simulink model "mainModel"  (R2025b)
settings: Solver=ode1  StartTime=0.0  StopTime=meas.u_alpha.time(end)  FixedStep=0.001  RelTol=1e-3
values from neighbouring files (symbols this model uses):
  alpha0 = params(1)    [Throttle_Parameter_Identification.m]
  alpha1 = params(2)    [Throttle_Parameter_Identification.m]
  R = 287    [Throttle_Parameter_Identification.m]
undefined symbols (not defined in the file or in its folder): beta0, gamma0, gamma1, H_l, k_eta, kappa, lambda, meas, nu0, nu1, nu_gen, sigma0, theta_e, Vc, Vd, Vm
settings Model: Creator=khanh  LastModifiedBy=khanh

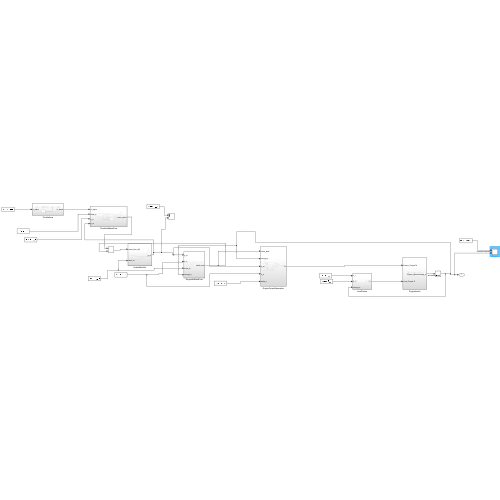
[thumbnail: Simulink's stored preview of the top-level diagram]
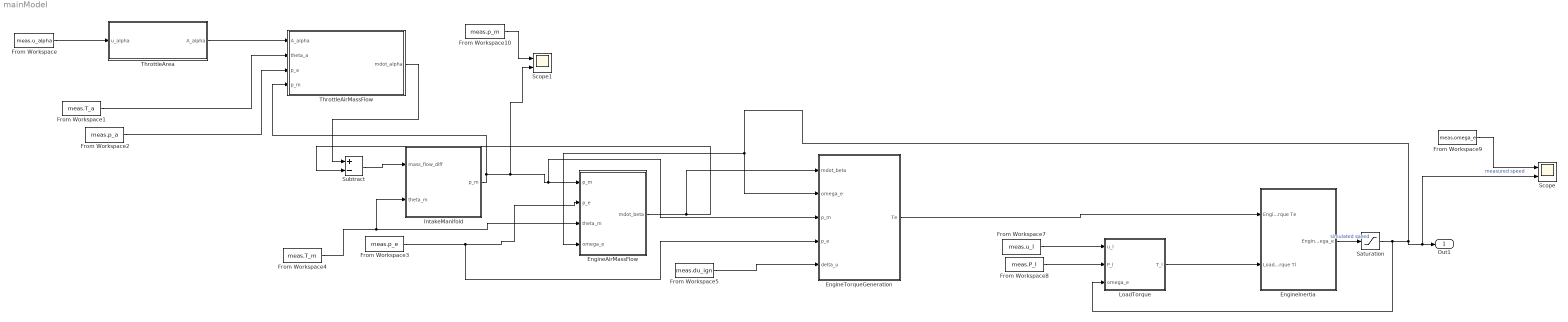
== system mainModel ==
  EngineAirMassFlow : Subsystem
  EngineInertia : Subsystem
  EngineTorqueGeneration : Subsystem
  From Workspace : FromWorkspace  VariableName=meas.u_alpha
  From Workspace1 : FromWorkspace  VariableName=meas.T_a
  From Workspace10 : FromWorkspace  VariableName=meas.p_m
  From Workspace2 : FromWorkspace  VariableName=meas.p_a
  From Workspace3 : FromWorkspace  VariableName=meas.p_e
  From Workspace4 : FromWorkspace  VariableName=meas.T_m
  From Workspace5 : FromWorkspace  VariableName=meas.du_ign
  From Workspace7 : FromWorkspace  VariableName=meas.u_l
  From Workspace8 : FromWorkspace  VariableName=meas.P_l
  From Workspace9 : FromWorkspace  VariableName=meas.omega_e
  IntakeManifold : Subsystem
  LoadTorque : Subsystem
  Saturation : Saturate  UpperLimit=500  LowerLimit=20
  Scope : Scope  NumInputPorts=2
      settings: ActiveDisplayYMinimum=-152.23064174316474  ActiveDisplayYMaximum=346.81367867125368
  Scope1 : Scope  NumInputPorts=2
      settings: ActiveDisplayYMinimum=10127.672299605907  ActiveDisplayYMaximum=44236.443903132655  DataLoggingVariableName=ScopeData4
  Subtract : Sum  Inputs=+-
  ThrottleAirMassFlow : Subsystem
  ThrottleArea : Subsystem
  Out1 : Outport
  wires:
  From Workspace2/1 -> ThrottleAirMassFlow/3(p_a)
  EngineAirMassFlow/1(mdot_beta) -> EngineTorqueGeneration/1(mdot_beta), Subtract/2
  From Workspace3/1 -> EngineTorqueGeneration/4(p_e), EngineAirMassFlow/2(p_e)
  From Workspace1/1 -> ThrottleAirMassFlow/2(theta_a)
  From Workspace4/1 -> EngineAirMassFlow/3(theta_m), IntakeManifold/2(theta_m)
  From Workspace/1 -> ThrottleArea/1(u_alpha)
  ThrottleArea/1(A_alpha) -> ThrottleAirMassFlow/1(A_alpha)
  ThrottleAirMassFlow/1(mdot_alpha) -> Subtract/1
  Saturation/1 -> LoadTorque/3(omega_e), Scope/2, Out1/1, EngineAirMassFlow/4(omega_e), EngineTorqueGeneration/2(omega_e)
  From Workspace9/1 -> Scope/1  "measured speed"
  LoadTorque/1(T_l) -> EngineInertia/2(Load_Torque Tl)
  From Workspace10/1 -> Scope1/1
  EngineTorqueGeneration/1(Te) -> EngineInertia/1(Engine_Torque Te)
  From Workspace7/1 -> LoadTorque/1(u_l)
  EngineInertia/1(Engine_Speed omega_e) -> Saturation/1  "simulated speed"
  Subtract/1 -> IntakeManifold/1(mass_flow_diff)
  From Workspace8/1 -> LoadTorque/2(P_l)
  From Workspace5/1 -> EngineTorqueGeneration/5(delta_u)
  IntakeManifold/1(p_m) -> ThrottleAirMassFlow/4(p_m), Scope1/2, EngineTorqueGeneration/3(p_m), EngineAirMassFlow/1(p_m)

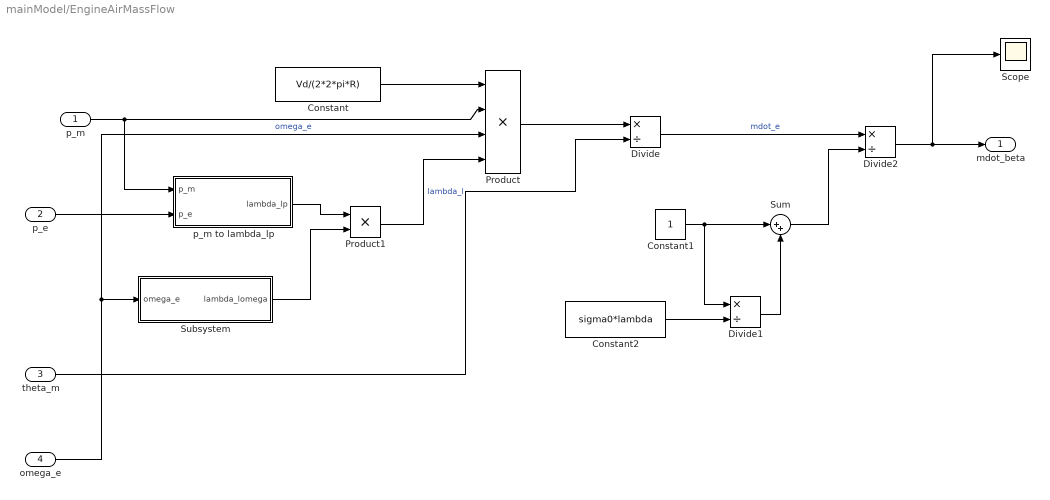
== system mainModel/EngineAirMassFlow ==
  p_m : Inport
  p_e : Inport  Port=2
  theta_m : Inport  Port=3
  omega_e : Inport  Port=4
  Constant : Constant  Value=Vd/(2*2*pi*R)
  Constant1 : Constant
  Constant2 : Constant  Value=sigma0*lambda
  Divide : Product  Inputs=*/
  Divide1 : Product  Inputs=*/
  Divide2 : Product  Inputs=*/
  Product : Product  Inputs=4
  Product1 : Product
  Scope : Scope
      settings: ActiveDisplayYMinimum=-1  ActiveDisplayYMaximum=1  DataLoggingVariableName=ScopeData3
  Subsystem : Subsystem
  Sum : Sum  Inputs=|++
  p_m to lambda_lp : Subsystem
  mdot_beta : Outport
  wires:
  Sum/1 -> Divide2/2
  Constant1/1 -> Divide1/1, Sum/1
  Divide/1 -> Divide2/1  "mdot_e"
  p_e/1 -> p_m to lambda_lp/2(p_e)
  Divide2/1 -> Scope/1, mdot_beta/1
  Constant/1 -> Product/1
  theta_m/1 -> Divide/2
  Product1/1 -> Product/4  "lambda_l"
  Constant2/1 -> Divide1/2
  omega_e/1 -> Product/3, Subsystem/1(omega_e)  "omega_e"
  Divide1/1 -> Sum/2
  p_m/1 -> p_m to lambda_lp/1(p_m), Product/2
  Product/1 -> Divide/1
  Subsystem/1(lambda_lomega) -> Product1/2
  p_m to lambda_lp/1(lambda_lp) -> Product1/1

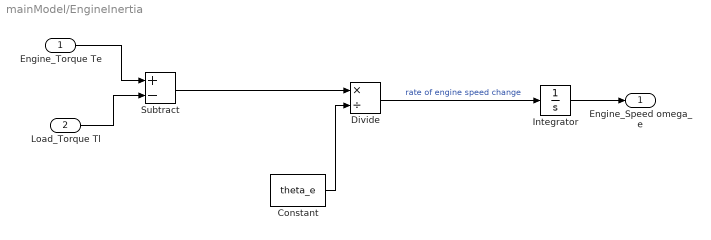
== system mainModel/EngineInertia ==
  Engine_Torque Te : Inport
  Load_Torque Tl : Inport  Port=2
  Constant : Constant  Value=theta_e
  Divide : Product  Inputs=*/
  Integrator : Integrator  InitialCondition=meas.omega_e.signals.values(1)
  Subtract : Sum  Inputs=+-
  Engine_Speed omega_e : Outport
  wires:
  Load_Torque Tl/1 -> Subtract/2
  Engine_Torque Te/1 -> Subtract/1
  Constant/1 -> Divide/2
  Divide/1 -> Integrator/1  "rate of engine speed change"
  Subtract/1 -> Divide/1
  Integrator/1 -> Engine_Speed omega_e/1

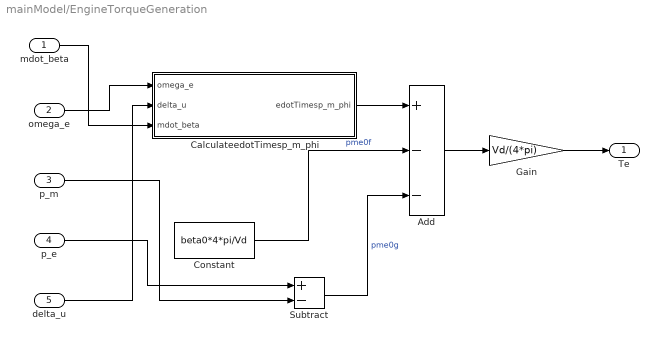
== system mainModel/EngineTorqueGeneration ==
  mdot_beta : Inport
  omega_e : Inport  Port=2
  p_m : Inport  Port=3
  p_e : Inport  Port=4
  delta_u : Inport  Port=5
  Add : Sum  Inputs=+--
  CalculateedotTimesp_m_phi : Subsystem
  Constant : Constant  Value=beta0*4*pi/Vd
  Gain : Gain  Gain=Vd/(4*pi)
  Subtract : Sum  Inputs=+-
  Te : Outport
  wires:
  Gain/1 -> Te/1
  Add/1 -> Gain/1
  Subtract/1 -> Add/3  "pme0g"
  p_m/1 -> Subtract/2
  delta_u/1 -> CalculateedotTimesp_m_phi/2(delta_u)
  CalculateedotTimesp_m_phi/1(edotTimesp_m_phi) -> Add/1
  mdot_beta/1 -> CalculateedotTimesp_m_phi/3(mdot_beta)
  Constant/1 -> Add/2  "pme0f"
  p_e/1 -> Subtract/1
  omega_e/1 -> CalculateedotTimesp_m_phi/1(omega_e)

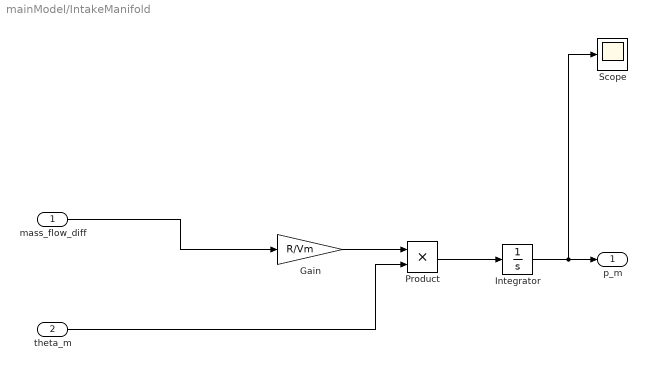
== system mainModel/IntakeManifold ==
  mass_flow_diff : Inport
  theta_m : Inport  Port=2
  Gain : Gain  Gain=R/Vm
  Integrator : Integrator  InitialCondition=meas.p_m.signals.values(1)
  Product : Product
  Scope : Scope
      settings: ActiveDisplayYMinimum=14149.965653298506  ActiveDisplayYMaximum=34149.96565329851  DataLoggingVariableName=ScopeData2
  p_m : Outport
  wires:
  Gain/1 -> Product/1
  Product/1 -> Integrator/1
  theta_m/1 -> Product/2
  Integrator/1 -> Scope/1, p_m/1
  mass_flow_diff/1 -> Gain/1

== system mainModel/LoadTorque ==
  u_l : Inport
  P_l : Inport  Port=2
  omega_e : Inport  Port=3
  Load Torque Subsystem : Subsystem
  T_l : Outport
  wires:
  P_l/1 -> Load Torque Subsystem/2(P_l)
  u_l/1 -> Load Torque Subsystem/1(u_l)
  omega_e/1 -> Load Torque Subsystem/3(omega_e)
  Load Torque Subsystem/1(Out1) -> T_l/1

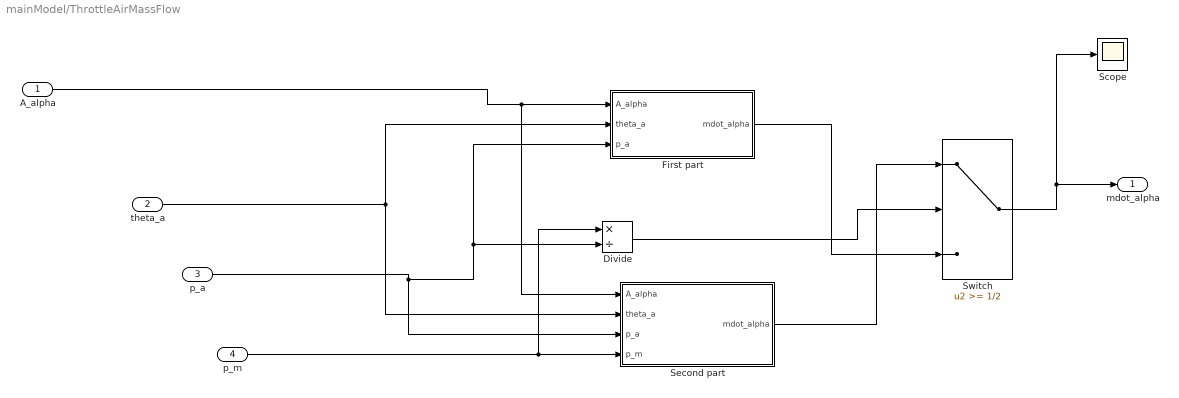
== system mainModel/ThrottleAirMassFlow ==
  A_alpha : Inport
  theta_a : Inport  Port=2
  p_a : Inport  Port=3
  p_m : Inport  Port=4
  Divide : Product  Inputs=*/
  First part : Subsystem
  Scope : Scope
      settings: ActiveDisplayYMinimum=-1  ActiveDisplayYMaximum=1
  "Second part " : Subsystem
  Switch : Switch  Threshold=1/2  SaturateOnIntegerOverflow=off  InputSameDT=off
  mdot_alpha : Outport
  wires:
  A_alpha/1 -> "Second part "/1(A_alpha), First part/1(A_alpha)
  p_a/1 -> "Second part "/3(p_a), First part/3(p_a), Divide/2
  p_m/1 -> "Second part "/4(p_m), Divide/1
  First part/1(mdot_alpha) -> Switch/3
  Switch/1 -> Scope/1, mdot_alpha/1
  Divide/1 -> Switch/2
  "Second part "/1(mdot_alpha) -> Switch/1
  theta_a/1 -> "Second part "/2(theta_a), First part/2(theta_a)

== system mainModel/ThrottleArea ==
  u_alpha : Inport
  Constant : Constant  Value=alpha0
  Gain : Gain  Gain=alpha1
  Sum : Sum  Inputs=|++
  A_alpha : Outport
  wires:
  Sum/1 -> A_alpha/1
  u_alpha/1 -> Gain/1
  Constant/1 -> Sum/2
  Gain/1 -> Sum/1

== system mainModel/EngineAirMassFlow/Subsystem ==
  omega_e : Inport
  Constant : Constant  Value=gamma0
  Gain : Gain  Gain=gamma1
  Sum : Sum  Inputs=|++
  lambda_lomega : Outport
  wires:
  Constant/1 -> Sum/1
  omega_e/1 -> Gain/1
  Gain/1 -> Sum/2
  Sum/1 -> lambda_lomega/1

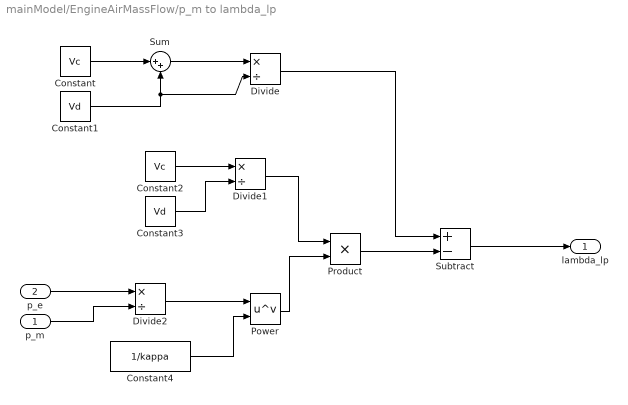
== system mainModel/EngineAirMassFlow/p_m to lambda_lp ==
  p_m : Inport
  p_e : Inport  Port=2
  Constant : Constant  Value=Vc
  Constant1 : Constant  Value=Vd
  Constant2 : Constant  Value=Vc
  Constant3 : Constant  Value=Vd
  Constant4 : Constant  Value=1/kappa
  Divide : Product  Inputs=*/
  Divide1 : Product  Inputs=*/
  Divide2 : Product  Inputs=*/
  Power : Math  Operator=pow
  Product : Product
  Subtract : Sum  Inputs=+-
  Sum : Sum  Inputs=|++
  lambda_lp : Outport
  wires:
  Constant/1 -> Sum/1
  Constant1/1 -> Sum/2, Divide/2
  Sum/1 -> Divide/1
  Constant2/1 -> Divide1/1
  Constant3/1 -> Divide1/2
  Divide2/1 -> Power/1
  Constant4/1 -> Power/2
  Divide1/1 -> Product/1
  Power/1 -> Product/2
  Divide/1 -> Subtract/1
  Product/1 -> Subtract/2
  Subtract/1 -> lambda_lp/1
  p_e/1 -> Divide2/1
  p_m/1 -> Divide2/2

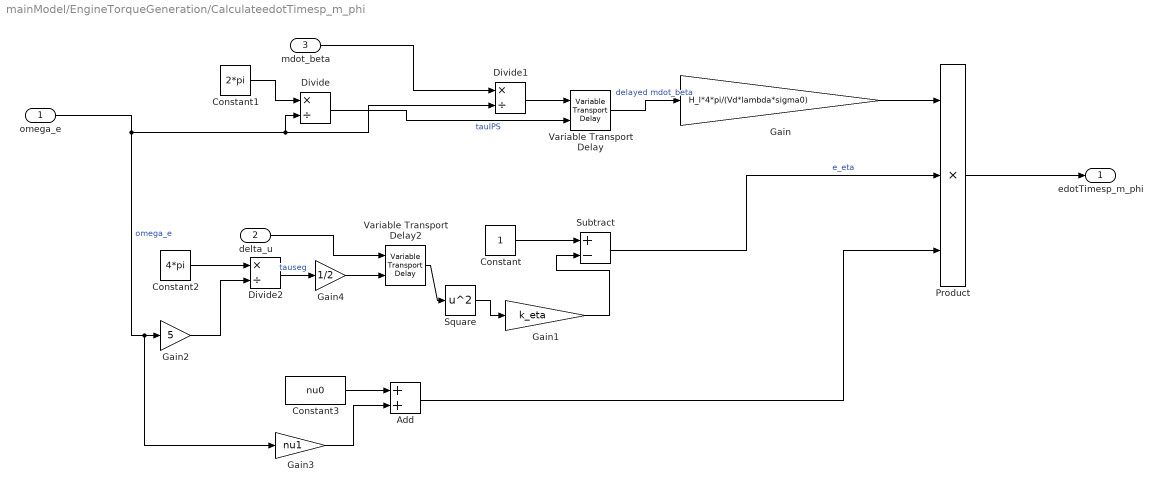
== system mainModel/EngineTorqueGeneration/CalculateedotTimesp_m_phi ==
  omega_e : Inport
  delta_u : Inport  Port=2
  mdot_beta : Inport  Port=3
  Add : Sum
  Constant : Constant
  Constant1 : Constant  Value=2*pi
  Constant2 : Constant  Value=4*pi
  Constant3 : Constant  Value=nu0
  Divide : Product  Inputs=*/
  Divide1 : Product  Inputs=*/
  Divide2 : Product  Inputs=*/
  Gain : Gain  Gain=H_l*4*pi/(Vd*lambda*sigma0)
  Gain1 : Gain  Gain=k_eta
  Gain2 : Gain  Gain=5
  Gain3 : Gain  Gain=nu1
  Gain4 : Gain  Gain=1/2
  Product : Product  Inputs=3
  Square : Math  Operator=square
  Subtract : Sum  Inputs=+-
  Variable Transport Delay : VariableTransportDelay  VariableDelayType=Variable transport delay  MaximumDelay=10
  Variable Transport Delay2 : VariableTransportDelay  VariableDelayType=Variable transport delay  MaximumDelay=10
  edotTimesp_m_phi : Outport
  wires:
  Constant/1 -> Subtract/1
  Gain1/1 -> Subtract/2
  Subtract/1 -> Product/2  "e_eta"
  omega_e/1 -> Gain3/1, Gain2/1, Divide1/2, Divide/2  "omega_e"
  Constant1/1 -> Divide/1
  Constant2/1 -> Divide2/1
  Gain2/1 -> Divide2/2
  Divide2/1 -> Gain4/1  "tauseg"
  delta_u/1 -> Variable Transport Delay2/1
  Constant3/1 -> Add/1
  Gain3/1 -> Add/2
  Gain/1 -> Product/1
  Add/1 -> Product/3
  Product/1 -> edotTimesp_m_phi/1
  Divide/1 -> Variable Transport Delay/2  "tauIPS"
  mdot_beta/1 -> Divide1/1
  Divide1/1 -> Variable Transport Delay/1
  Variable Transport Delay/1 -> Gain/1  "delayed mdot_beta"
  Variable Transport Delay2/1 -> Square/1
  Square/1 -> Gain1/1
  Gain4/1 -> Variable Transport Delay2/2

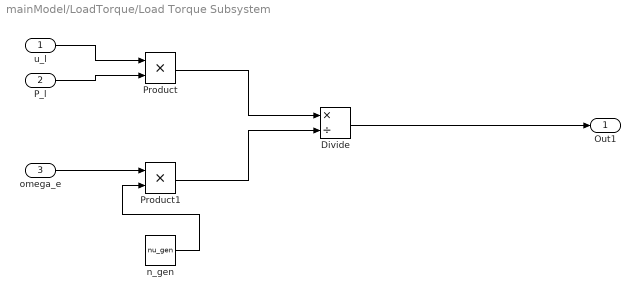
== system mainModel/LoadTorque/Load Torque Subsystem ==
  u_l : Inport
  P_l : Inport  Port=2
  omega_e : Inport  Port=3
  Divide : Product  Inputs=*/
  Product : Product
  Product1 : Product
  n_gen : Constant  Value=nu_gen
  Out1 : Outport
  wires:
  P_l/1 -> Product/2
  u_l/1 -> Product/1
  omega_e/1 -> Product1/1
  n_gen/1 -> Product1/2
  Divide/1 -> Out1/1
  Product/1 -> Divide/1
  Product1/1 -> Divide/2

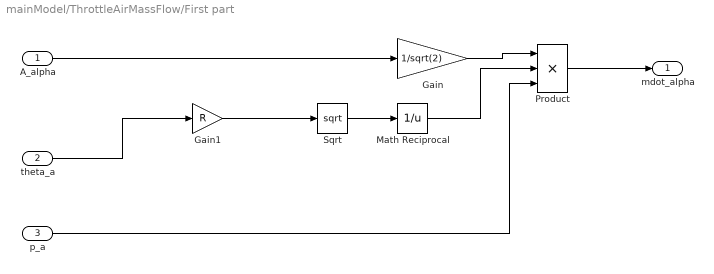
== system mainModel/ThrottleAirMassFlow/First part ==
  A_alpha : Inport
  theta_a : Inport  Port=2
  p_a : Inport  Port=3
  Gain : Gain  Gain=1/sqrt(2)
  Gain1 : Gain  Gain=R
  Math Reciprocal : Math  Operator=reciprocal  SignedPower=on
  Product : Product  Inputs=3
  Sqrt : Sqrt
  mdot_alpha : Outport
  wires:
  Sqrt/1 -> Math Reciprocal/1
  p_a/1 -> Product/3
  Gain/1 -> Product/1
  Gain1/1 -> Sqrt/1
  theta_a/1 -> Gain1/1
  Product/1 -> mdot_alpha/1
  A_alpha/1 -> Gain/1
  Math Reciprocal/1 -> Product/2

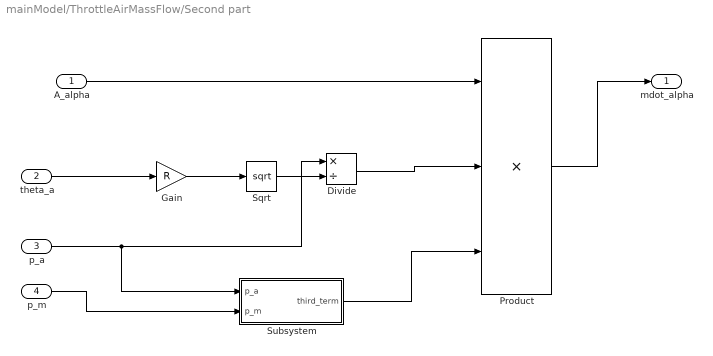
== system mainModel/ThrottleAirMassFlow/Second part  ==
  A_alpha : Inport
  theta_a : Inport  Port=2
  p_a : Inport  Port=3
  p_m : Inport  Port=4
  Divide : Product  Inputs=*/
  Gain : Gain  Gain=R
  Product : Product  Inputs=3
  Sqrt : Sqrt
  Subsystem : Subsystem
  mdot_alpha : Outport
  wires:
  Product/1 -> mdot_alpha/1
  A_alpha/1 -> Product/1
  theta_a/1 -> Gain/1
  Gain/1 -> Sqrt/1
  Sqrt/1 -> Divide/2
  p_a/1 -> Subsystem/1(p_a), Divide/1
  Divide/1 -> Product/2
  p_m/1 -> Subsystem/2(p_m)
  Subsystem/1(third_term) -> Product/3

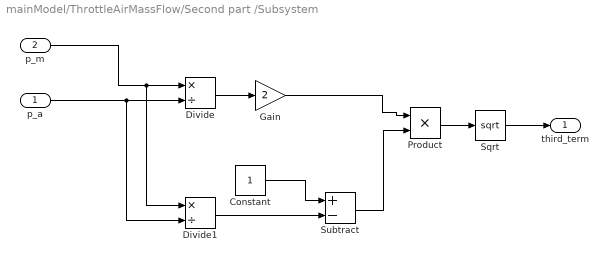
== system mainModel/ThrottleAirMassFlow/Second part /Subsystem ==
  p_a : Inport
  p_m : Inport  Port=2
  Constant : Constant
  Divide : Product  Inputs=*/
  Divide1 : Product  Inputs=*/
  Gain : Gain  Gain=2
  Product : Product
  Sqrt : Sqrt
  Subtract : Sum  Inputs=+-
  third_term : Outport
  wires:
  Divide/1 -> Gain/1
  p_a/1 -> Divide1/2, Divide/2
  p_m/1 -> Divide1/1, Divide/1
  Divide1/1 -> Subtract/2
  Constant/1 -> Subtract/1
  Gain/1 -> Product/1
  Subtract/1 -> Product/2
  Product/1 -> Sqrt/1
  Sqrt/1 -> third_term/1
